simulink model "Real_World_Rotate_270"  (R2021a)
settings: Solver=VariableStepAuto  StartTime=0.0  StopTime=10.0  RelTol=1e-3
values from neighbouring files (symbols this model uses):
  axleLength = 0.136    [robotParameters.m]
  ticksPerRot = 20    [robotParameters.m]
  wheelR = 0.031    [robotParameters.m]
undefined symbols (not defined in the file or in its folder): InputPWM, WheelSpeed
libraries: arduinolib x4, spsEdgeDetectorLib x2, mobileRoboticsTrainingLib x1
settings Model: Creator=akhil  LastModifiedBy=akhil

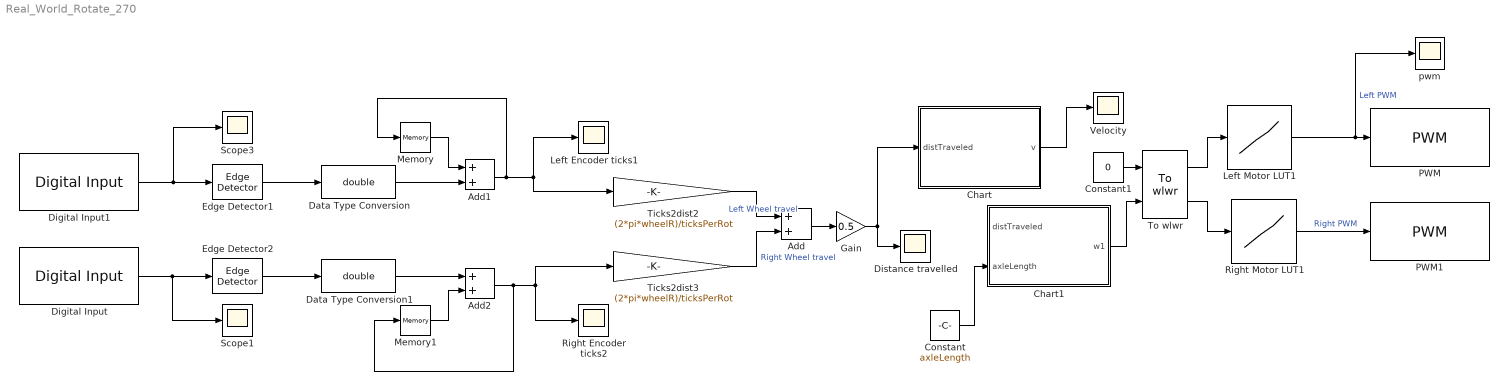
== system Real_World_Rotate_270 ==
  Add : Sum
  Add1 : Sum
  Add2 : Sum
  Chart : Stateflow chart  TreatAsAtomicUnit=on
  Chart1 : Stateflow chart  TreatAsAtomicUnit=on
  Constant : Constant  Value=axleLength
  Constant1 : Constant  Value=0
  Data Type Conversion : DataTypeConversion  OutDataTypeStr=double
  Data Type Conversion1 : DataTypeConversion  OutDataTypeStr=double
  Digital Input : arduinolib/Digital Input  pinNumber=3  mode=Default  Direction=input  SampleTime=0.01  blockPlatform=arduino
  Digital Input1 : arduinolib/Digital Input  pinNumber=2  mode=Default  Direction=input  SampleTime=0.01  blockPlatform=arduino
  Distance travelled : Scope
  Edge Detector1 : spsEdgeDetectorLib/Edge Detector  model=Rising  ic=0  Ts=0
      settings: SourceProductBaseCode=PS
  Edge Detector2 : spsEdgeDetectorLib/Edge Detector  model=Rising  ic=0  Ts=0
      settings: SourceProductBaseCode=PS
  Gain : Gain  Gain=0.5
  Left Encoder ticks1 : Scope
  Left Motor LUT1 : Lookup_n-D  NumberOfTableDimensions=1  BreakpointsForDimension1=WheelSpeed  Table=InputPWM  InterpMethod=Nearest  ExtrapMethod=Clip  InternalRulePriority=Speed  RndMeth=Simplest  InputSameDT=on
  Memory : Memory
  Memory1 : Memory
  PWM : arduinolib/PWM  pinNumber=5  frequencyType=Default  desiredFrequency=490.2  achievableFrequency=490.2
  PWM1 : arduinolib/PWM  pinNumber=6  frequencyType=Default  desiredFrequency=490.2  achievableFrequency=490.2
  Right Encoder ticks2 : Scope
  Right Motor LUT1 : Lookup_n-D  NumberOfTableDimensions=1  BreakpointsForDimension1=WheelSpeed  Table=InputPWM  InterpMethod=Nearest  ExtrapMethod=Clip  InternalRulePriority=Speed  RndMeth=Simplest  InputSameDT=on
  Scope1 : Scope
  Scope3 : Scope
  Ticks2dist2 : Gain  Gain=(2*pi*wheelR)/ticksPerRot
  Ticks2dist3 : Gain  Gain=(2*pi*wheelR)/ticksPerRot
  To wlwr : mobileRoboticsTrainingLib/To wlwr  axleLength=0.1  wheelR=0.05
  Velocity : Scope
  pwm : Scope
  wires:
  Chart1/1(w1) -> To wlwr/2
  Add/1 -> Gain/1
  Edge Detector1/1 -> Data Type Conversion/1
  Constant/1 -> Chart1/2(axleLength)
  Gain/1 -> Chart/1(distTraveled), Distance travelled/1
  To wlwr/1 -> Left Motor LUT1/1
  Data Type Conversion1/1 -> Add2/1
  Add1/1 -> Memory/1, Ticks2dist2/1, Left Encoder ticks1/1
  Add2/1 -> Memory1/1, Ticks2dist3/1, Right Encoder ticks2/1
  Digital Input/1 -> Scope1/1, Edge Detector2/1
  Data Type Conversion/1 -> Add1/2
  Edge Detector2/1 -> Data Type Conversion1/1
  Right Motor LUT1/1 -> PWM1/1  "Right PWM"
  Chart/1(v) -> Velocity/1
  Digital Input1/1 -> Scope3/1, Edge Detector1/1
  To wlwr/2 -> Right Motor LUT1/1
  Memory1/1 -> Add2/2
  Constant1/1 -> To wlwr/1
  Memory/1 -> Add1/1
  Left Motor LUT1/1 -> pwm/1, PWM/1  "Left PWM"
  Ticks2dist3/1 -> Add/2  "Right Wheel travel"
  Ticks2dist2/1 -> Add/1  "Left Wheel travel"

== stateflow chart Real_World_Rotate_270/Chart1 ==
  state For 90°: pi/2 [commented out]
    For 180°: pi
    for 270°: 3*pi/2
    For 360°: 2*pi
  state Rotate
    entry:
    w1=pi/6
    %wl = -0.55
    %wr = 0.55
  state Stop
    entry:
    w1=0
    %wl = 0
    %wr = 0
  (default) -> Rotate : % Start
  Rotate -> Stop : [2*distTraveled/axleLength >= 3*pi/2]
  Stop -> Rotate : [2*distTraveled/axleLength < 3*pi/2]
  data: distTraveled input; axleLength input; w1 output

== stateflow chart Real_World_Rotate_270/Chart ==
  state MoveForward
    entry:
    v = 0.1
  state Stop
    entry:
    v = 0
  (default) -> MoveForward : % Start
  MoveForward -> Stop : [distTraveled >= 1]
  data: distTraveled input; v output
